simulink model "OuterLoop_Control_Harness_HLR_6"  (R2024a)
settings: Solver=FixedStepDiscrete  StartTime=0.0  StopTime=10.0  RelTol=1e-3  EnableMultiTasking=on
settings Model: DataDictionary=DD_OuterLoop_Control.sldd  Creator=The MathWorks, Inc.  LastModifiedBy=The MathWorks, Inc.
settings SolverCC: AlgebraicLoopSolver=TrustRegion  MaxZcPerStep=1
settings DataIOCC: LimitDataPoints=on
settings OptimizationCC: BlockReduction=off  DefaultParameterBehavior=Inlined  UseDivisionForNetSlopeComputation=on  UseFloatMulNetSlope=on  InlineInvariantSignals=on  EnhancedBackFolding=on  PassReuseOutputArgsAs=Individual arguments  EfficientFloat2IntCast=on  EfficientMapNaN2IntZero=off  LifeSpan=inf  MaxStackSize=inf  OptimizeBlockOrder=speed  EfficientTunableParamExpr=on
settings DebuggingCC: SignalInfNanChecking=error  SignalRangeChecking=error  ReadBeforeWriteMsg=EnableAllAsError  WriteAfterWriteMsg=EnableAllAsError  WriteAfterReadMsg=EnableAllAsError  AlgebraicLoopMsg=error  ArtificialAlgebraicLoopMsg=error  SaveWithDisabledLinksMsg=error  SaveWithParameterizedLinksMsg=error  BlockPriorityViolationMsg=error  SolverPrmCheckMsg=error  InheritedTsInSrcMsg=error  SingleTaskRateTransMsg=error  TasksWithSamePriorityMsg=error  SigSpecEnsureSampleTimeMsg=error  CheckMatrixSingularityMsg=error  IntegerOverflowMsg=error  ParameterUnderflowMsg=error  ParameterPrecisionLossMsg=error  ParameterTunabilityLossMsg=error  UnderSpecifiedDataTypeMsg=error  UnnecessaryDatatypeConvMsg=warning  VectorMatrixConversionMsg=error  SignalLabelMismatchMsg=error  UnconnectedInputMsg=error  UnconnectedOutputMsg=error  UnconnectedLineMsg=error  SFcnCompatibilityMsg=error  UniqueDataStoreMsg=error  BusObjectLabelMismatch=error  RootOutportRequireBusObject=error  AssertControl=DisableAll  AllowSymbolicDim=off  ModelReferenceIOMismatchMessage=error  UnknownTsInhSupMsg=error  ModelReferenceDataLoggingMessage=error  ModelReferenceSymbolNameMessage=none  StateNameClashWarn=warning  PregeneratedLibrarySubsystemCodeDiagnostic=none  StrictBusMsg=ErrorOnBusTreatedAsVector  NonBusSignalsTreatedAsBus=error  SFInvalidInputDataAccessInChartInitDiag=error  SFTransitionOutsideNaturalParentDiag=error  SFUnreachableExecutionPathDiag=error  SFUndirectedBroadcastEventsDiag=error  SFTransitionActionBeforeConditionDiag=error  SFExecutionAtInitializationDiag=none  IntegerSaturationMsg=error  ArithmeticOperatorsInVariantConditions=warning
settings HardwareCC: ProdBitPerPointer=32  ProdBitPerSizeT=32  ProdBitPerPtrDiffT=32  ProdLargestAtomicInteger=Long  ProdWordSize=32  ProdHWDeviceType=ARM Compatible->ARM 10
settings ModelReferenceCC: EnableRefExpFcnMdlSchedulingChecks=on  ModelReferenceNumInstancesAllowed=Single  PropagateSignalLabelsOutOfModel=off
settings SFSimCC: CompileTimeRecursionLimit=0  EnableRuntimeRecursion=off  MATLABDynamicMemAlloc=off  CustomCodeUndefinedFunction=UseInterfaceOnly
settings RTWCC: Description=Embedded Coder  SystemTargetFile=ert.tlc  GenCodeOnly=on  TemplateMakefile=ert_default_tmf  GenerateReport=on  BuildConfiguration=Faster Runs  IncludeHyperlinkInReport=on  LaunchReport=on  GenerateTraceInfo=on  GenerateTraceReport=on  GenerateTraceReportSl=on  GenerateTraceReportSf=on  GenerateTraceReportEml=on  GenerateCodeMetricsReport=on  GPUComputeCapability=3.5  DLArmComputeVersion=19.05
settings CodeAppCC: ForceParamTrailComments=on  IgnoreCustomStorageClasses=off  MATLABFcnDesc=on  MangleLength=4  StateflowObjectComments=on  ReqsInCode=on
settings ERTTargetCC: TargetLangStandard=C99 (ISO)  UtilityFuncGeneration=Shared location  GenerateSampleERTMain=on  IncludeMdlTerminateFcn=off  SuppressErrorStatus=on  SupportAbsoluteTime=off  SupportNonFinite=off  RemoveDisableFunc=on  ParenthesesLevel=Maximum  CastingMode=Standards  GenerateSharedConstants=off  InlinedParameterPlacement=NonHierarchical  ERTCustomFileTemplate=example_file_process.tlc  PreserveExpressionOrder=on  PreserveIfCondition=on  SuppressUnreachableDefaultCases=off  EnableSignedLeftShifts=off  EnableSignedRightShifts=off
settings ConfigComp: CovAccelSimSupport=on

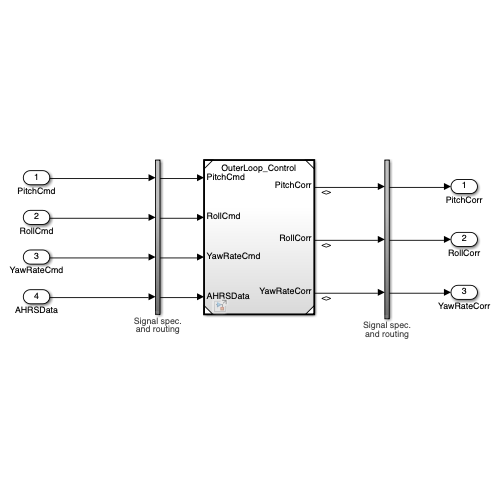
[thumbnail: Simulink's stored preview of the top-level diagram]
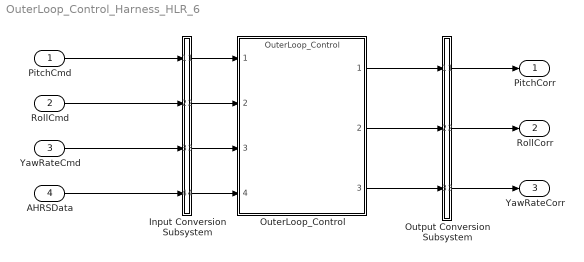
== system OuterLoop_Control_Harness_HLR_6 ==
  PitchCmd : Inport  OutDataTypeStr=double  PortDimensions=[1]  SampleTime=0.01
  RollCmd : Inport  Port=2  OutDataTypeStr=double  PortDimensions=[1]  SampleTime=0.01
  YawRateCmd : Inport  Port=3  OutDataTypeStr=double  PortDimensions=[1]  SampleTime=0.01
  AHRSData : Inport  Port=4  OutDataTypeStr=double  PortDimensions=[5]  SampleTime=0.01
  Input Conversion Subsystem : Subsystem  Tag=__SLT_ICS__  Description=|
      | Signal spec.
      | and routing
      settings: AttributesFormatString=%<Description>
  OuterLoop_Control : ModelReference  ModelNameDialog=OuterLoop_Control  SimulationMode=Normal  ModelReferenceVersion=3.0
  Output Conversion Subsystem : Subsystem  Tag=__SLT_OCS__  Description=|
      | Signal spec.
      | and routing
      settings: AttributesFormatString=%<Description>
  PitchCorr : Outport
  RollCorr : Outport  Port=2
  YawRateCorr : Outport  Port=3
  wires:
  PitchCmd/1 -> Input Conversion Subsystem/1(Inport_1)
  RollCmd/1 -> Input Conversion Subsystem/2(Inport_2)
  YawRateCmd/1 -> Input Conversion Subsystem/3(Inport_3)
  AHRSData/1 -> Input Conversion Subsystem/4(Inport_4)
  Output Conversion Subsystem/1(Outport_1) -> PitchCorr/1
  Output Conversion Subsystem/2(Outport_2) -> RollCorr/1
  Output Conversion Subsystem/3(Outport_3) -> YawRateCorr/1
  Input Conversion Subsystem/1(Outport_1) -> OuterLoop_Control/1
  Input Conversion Subsystem/2(Outport_2) -> OuterLoop_Control/2
  Input Conversion Subsystem/3(Outport_3) -> OuterLoop_Control/3
  Input Conversion Subsystem/4(Outport_4) -> OuterLoop_Control/4
  OuterLoop_Control/1 -> Output Conversion Subsystem/1(Inport_1)
  OuterLoop_Control/2 -> Output Conversion Subsystem/2(Inport_2)
  OuterLoop_Control/3 -> Output Conversion Subsystem/3(Inport_3)

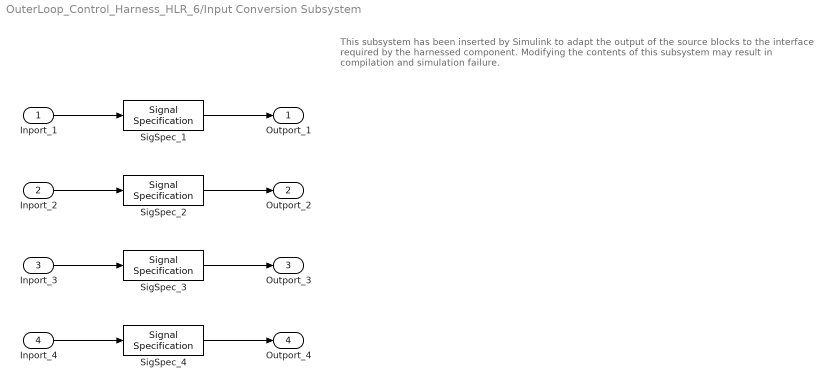
== system OuterLoop_Control_Harness_HLR_6/Input Conversion Subsystem ==
  note: This subsystem has been inserted by Simulink to adapt the output of the source blocks to the interface required by the harnessed component.
      |  Modifying the contents of this subsystem may result in compilation and simulation failure.
  Inport_1 : Inport
  Inport_2 : Inport  Port=2
  Inport_3 : Inport  Port=3
  Inport_4 : Inport  Port=4
  SigSpec_1 : SignalSpecification  OutDataTypeStr=double  Dimensions=[1]  SampleTime=0.01
  SigSpec_2 : SignalSpecification  OutDataTypeStr=double  Dimensions=[1]  SampleTime=0.01
  SigSpec_3 : SignalSpecification  OutDataTypeStr=double  Dimensions=[1]  SampleTime=0.01
  SigSpec_4 : SignalSpecification  OutDataTypeStr=double  Dimensions=[5]  SampleTime=0.01
  Outport_1 : Outport
  Outport_2 : Outport  Port=2
  Outport_3 : Outport  Port=3
  Outport_4 : Outport  Port=4
  wires:
  SigSpec_1/1 -> Outport_1/1
  Inport_1/1 -> SigSpec_1/1
  SigSpec_2/1 -> Outport_2/1
  Inport_2/1 -> SigSpec_2/1
  SigSpec_3/1 -> Outport_3/1
  Inport_3/1 -> SigSpec_3/1
  SigSpec_4/1 -> Outport_4/1
  Inport_4/1 -> SigSpec_4/1

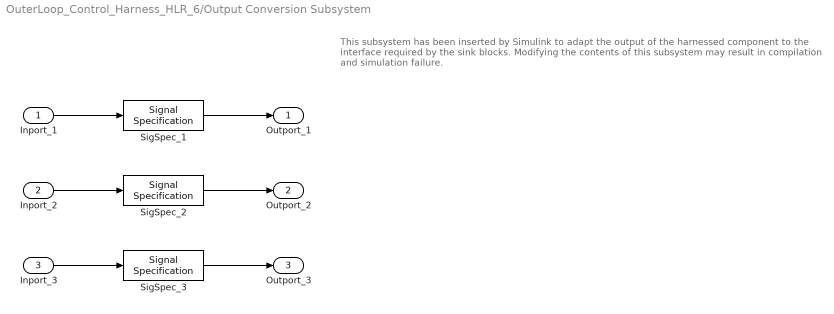
== system OuterLoop_Control_Harness_HLR_6/Output Conversion Subsystem ==
  note: This subsystem has been inserted by Simulink to adapt the output of the harnessed component to the interface required by the sink blocks.
      |  Modifying the contents of this subsystem may result in compilation and simulation failure.
  Inport_1 : Inport
  Inport_2 : Inport  Port=2
  Inport_3 : Inport  Port=3
  SigSpec_1 : SignalSpecification  OutDataTypeStr=double  Dimensions=[1]  SampleTime=0.01
  SigSpec_2 : SignalSpecification  OutDataTypeStr=double  Dimensions=[1]  SampleTime=0.01
  SigSpec_3 : SignalSpecification  OutDataTypeStr=double  Dimensions=[1]  SampleTime=0.01
  Outport_1 : Outport
  Outport_2 : Outport  Port=2
  Outport_3 : Outport  Port=3
  wires:
  Inport_1/1 -> SigSpec_1/1
  SigSpec_1/1 -> Outport_1/1
  Inport_2/1 -> SigSpec_2/1
  SigSpec_2/1 -> Outport_2/1
  Inport_3/1 -> SigSpec_3/1
  SigSpec_3/1 -> Outport_3/1
